simulink model "Micro_Grid_Mains_OFF"  (R2024b)
settings: Solver=VariableStepAuto  StartTime=0.0  StopTime=60*3  RelTol=1e-3
values from neighbouring files (symbols this model uses):
  Pref = 1    [MicroGridParameters.m]
  Ts = 30e-6    (= 3e-05)    [MicroGridParameters.m]
  VDC_Link = 12    [MicroGridParameters.m]
  Vref = 200    [MicroGridParameters.m]
  wref = 1    [MicroGridParameters.m]
libraries: spsSeriesRLCBranchLib x9, spsVoltageMeasurementLib x9, spsThreePhaseVIMeasurementLib x6, spsThreePhaseSeriesRLCBranchLib x5, spsThreePhaseSourceLib x3, spsDiodeLib x3, spsMosfetLib x3, spsPWMGeneratorDCDCLib x3, spsThreePhaseSeriesRLCLoadLib x2, spsBreakerLib x2, spsUniversalBridgeLib x2, slpidlib x2
settings Model: SimulationMode=accelerator  Creator=haima  LastModifiedBy=haima

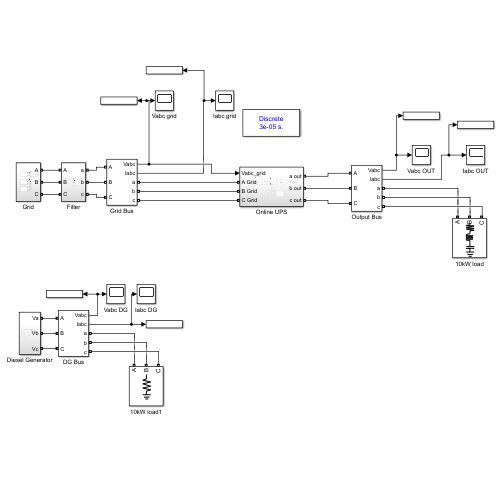
[thumbnail: Simulink's stored preview of the top-level diagram]
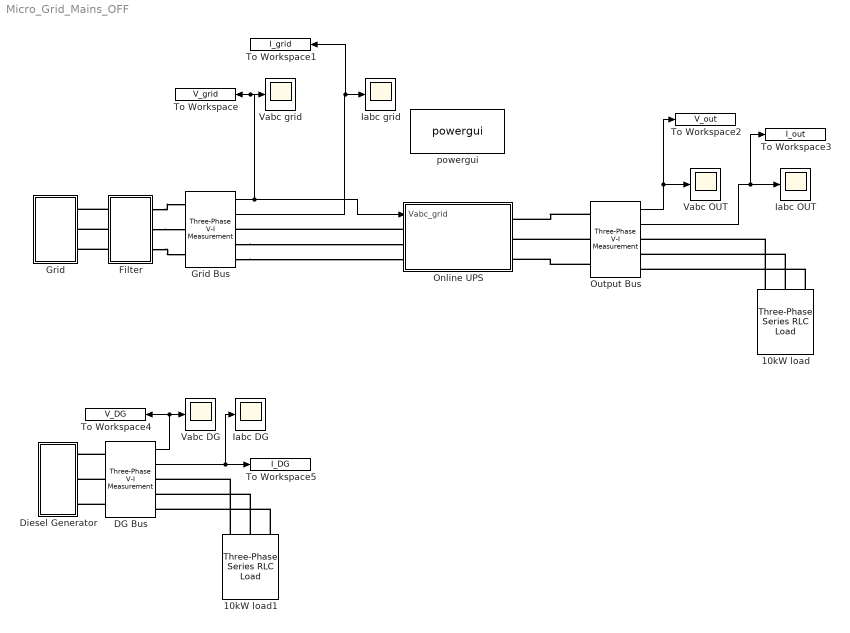
== system Micro_Grid_Mains_OFF ==
  10kW load : spsThreePhaseSeriesRLCLoadLib/Three-Phase Series RLC Load  LConnTagsString=A|B|C  Configuration=Y (grounded)  NominalVoltage=1000  Vabc=[1e3 1e3 1e3]  Vabcp=[1e3 1e3 1e3]  NominalFrequency=50  UnbalancedPower=off  ActivePower=10e3  InductivePower=100  CapacitivePower=100  Pabc=[10e3 9e3 11e3]  QLabc=[100 90 110]  QCabc=[100 90 110]  Pabcp=[10e3 9e3 11e3]  QLabcp=[100 90 110]  QCabcp=[100 90 110]  Measurements=None  LoadType=constant Z
  10kW load1 : spsThreePhaseSeriesRLCLoadLib/Three-Phase Series RLC Load  LConnTagsString=A|B|C  Configuration=Y (grounded)  NominalVoltage=1000  Vabc=[1e3 1e3 1e3]  Vabcp=[1e3 1e3 1e3]  NominalFrequency=50  UnbalancedPower=off  ActivePower=10e3  InductivePower=0  CapacitivePower=0  Pabc=[10e3 9e3 11e3]  QLabc=[100 90 110]  QCabc=[100 90 110]  Pabcp=[10e3 9e3 11e3]  QLabcp=[100 90 110]  QCabcp=[100 90 110]  Measurements=None  LoadType=constant Z
  DG Bus : spsThreePhaseVIMeasurementLib/Three-Phase V-I Measurement  VoltageMeasurement=phase-to-ground  SetLabelV=off  LabelV=Vabc  Vpu=off  VpuLL=off  CurrentMeasurement=yes  SetLabelI=off  LabelI=Iabc  Ipu=off  Pbase=100e6  Vbase=500e3  OutputType=Complex  PhasorSimulation=off  PSBequivalent=0
  Diesel Generator : Subsystem
  Filter : Subsystem
  Grid : Subsystem
  Grid Bus : spsThreePhaseVIMeasurementLib/Three-Phase V-I Measurement  VoltageMeasurement=phase-to-ground  SetLabelV=off  LabelV=Vabc  Vpu=off  VpuLL=off  CurrentMeasurement=yes  SetLabelI=off  LabelI=Iabc  Ipu=off  Pbase=100e6  Vbase=500e3  OutputType=Complex  PhasorSimulation=off  PSBequivalent=0
  Iabc DG : Scope
  Iabc OUT : Scope
  Iabc grid : Scope
  Online UPS : Subsystem
  Output Bus : spsThreePhaseVIMeasurementLib/Three-Phase V-I Measurement  VoltageMeasurement=phase-to-ground  SetLabelV=off  LabelV=Vabc  Vpu=off  VpuLL=off  CurrentMeasurement=yes  SetLabelI=off  LabelI=Iabc  Ipu=off  Pbase=100e6  Vbase=500e3  OutputType=Complex  PhasorSimulation=off  PSBequivalent=0
  To Workspace : ToWorkspace  VariableName=V_grid  SaveFormat=Timeseries  SampleTime=-1
  To Workspace1 : ToWorkspace  VariableName=I_grid  SaveFormat=Timeseries  SampleTime=-1
  To Workspace2 : ToWorkspace  VariableName=V_out  SaveFormat=Timeseries  SampleTime=-1
  To Workspace3 : ToWorkspace  VariableName=I_out  SaveFormat=Timeseries  SampleTime=-1
  To Workspace4 : ToWorkspace  VariableName=V_DG  SaveFormat=Timeseries  SampleTime=-1
  To Workspace5 : ToWorkspace  VariableName=I_DG  SaveFormat=Timeseries  SampleTime=-1
  Vabc DG : Scope
  Vabc OUT : Scope
  Vabc grid : Scope
  powergui : spspowerguiLib/powergui  SimulationMode=Discrete  SampleTime=Ts  frequency=60  Iterations=50  frequencyindice=50  Pbase=100e6  ErrMax=1e-4  UnitsV=kV  UnitsW=MW  buscounter=0  FunctionMessages=off  echomessages=off  EnableUseOfTLC=off  CurrentSourceSwitches=off  DisableSnubberDevices=off  DisableRonSwitches=off  DisableVfSwitches=off  DisplayEquations=off  AutomaticDiscreteSolvers=off  SolverType=Tustin/Backward Euler (TBE)  Interpol=off  ExternalGateDelay=off  methode=off  Ts=100  x0status=blocks  SPID=off  SwTol=0  HookPort=off  NonlinearTolerance=1e-4  nMaxIteration=100  ContinueOnMaxIteration=off  RestoreLinks=warning  ResistiveCurrentMeasurement=off  Frange=[0:2:500]  Ylog=off  Xlog=on  ShowGrid=off  save=off  variable=ZData  structure=Outputs  ZoomFFT=off  StartTime=0.07  cycles=2  DisplayStyle=1  fundamental=50  FreqAxis=on  MaxFrequency=2000  frequencyindicesteady=1  RmsSteady=2  display=off
  wires:
  Grid Bus/1 -> Online UPS/1(Vabc_grid), Vabc grid/1, To Workspace/1
  Grid Bus/2 -> To Workspace1/1, Iabc grid/1
  DG Bus/1 -> Vabc DG/1, To Workspace4/1
  DG Bus/2 -> To Workspace5/1, Iabc DG/1
  Output Bus/1 -> To Workspace2/1, Vabc OUT/1
  Output Bus/2 -> To Workspace3/1, Iabc OUT/1
  connections:
  DG Bus/LConn2 -- Diesel Generator/RConn2
  DG Bus/LConn1 -- Diesel Generator/RConn1
  DG Bus/LConn3 -- Diesel Generator/RConn3
  Output Bus/LConn1 -- Online UPS/RConn1
  Output Bus/LConn2 -- Online UPS/RConn2
  Output Bus/LConn3 -- Online UPS/RConn3
  Filter/LConn1 -- Grid/RConn1
  Filter/LConn2 -- Grid/RConn2
  Filter/LConn3 -- Grid/RConn3
  Filter/RConn2 -- Grid Bus/LConn2
  Filter/RConn1 -- Grid Bus/LConn1
  Filter/RConn3 -- Grid Bus/LConn3
  10kW load/LConn1 -- Output Bus/RConn1
  10kW load/LConn2 -- Output Bus/RConn2
  10kW load/LConn3 -- Output Bus/RConn3
  Online UPS/LConn1 -- Grid Bus/RConn1
  Grid Bus/RConn2 -- Online UPS/LConn2
  Grid Bus/RConn3 -- Online UPS/LConn3
  10kW load1/LConn1 -- DG Bus/RConn1
  10kW load1/LConn2 -- DG Bus/RConn2
  10kW load1/LConn3 -- DG Bus/RConn3

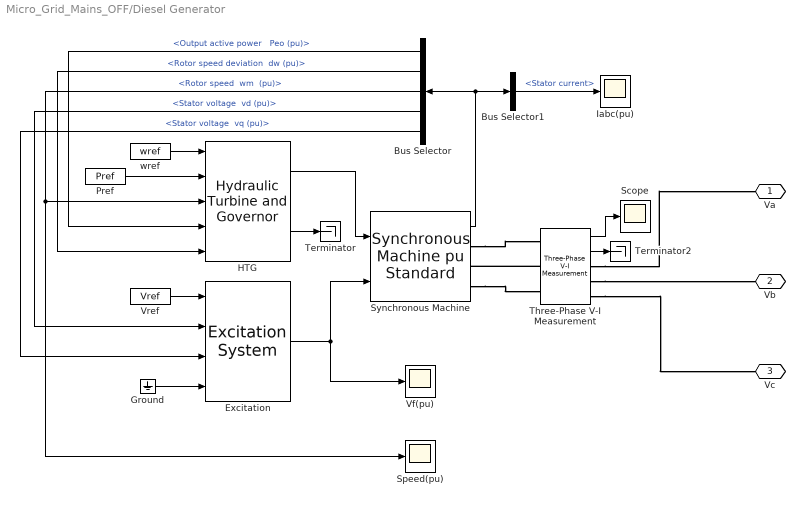
== system Micro_Grid_Mains_OFF/Diesel Generator ==
  Bus Selector : BusSelector  OutputSignals="Output active power   Peo (pu),Mechanical.Rotor speed deviation  dw (pu),Mechanical.Rotor speed  wm  (pu),dq0 components.Stator voltage  vd (pu),dq0 components.Stator voltage  vq (pu)"
  Bus Selector1 : BusSelector  OutputSignals=Stator current
  "Excitation " : spsExcitationSystemLib/Excitation System  tr=20e-3  reg=[ 300, 0.001 ]  exc=[ 1, 0 ]  tgr=[ 0, 0 ]  damp=[ 0.001, 0.1 ]  sat=[ 0, 0 ]  lim=[ -11.5, 11.5, 0 ]  v0="[1.0  1.28]"
  Ground : Ground
  HTG : spsHydraulicTurbineandGovernorLib/Hydraulic Turbine and Governor  sm="[ 10/3  0.07 ]"  gate="[  0.01  0.97518  -0.1  0.1 ]"  reg="[  0.05  1.163  0.105  0  0.01  ]"  hyd="[  0  2.67  ]"  dref=0  po=0.400114
  Iabc(pu) : Scope
  Pref : Constant  Value=Pref
  Scope : Scope
  Speed(pu) : Scope
  "Synchronous Machine " : spsSynchronousMachinepuStandardLib/Synchronous Machine pu Standard  PresetModel=No  MechanicalLoad=Mechanical power Pm  ShowDetailedParameters=on  RotorType=Salient-pole  Units=per unit standard parameters  MeasurementBus=off  NominalParameters=PowerVoltageFrequency  Reactances1=[ 1.81, 0.3, 0.23, 1.76, 0.65, 0.25, 0.15 ]  Reactances2=Reactances  dAxisTimeConstants=Short-circuit  qAxisTimeConstants=Short-circuit  TimeConstants1="[ 4.4849  0.0681  0.1  ]"  TimeConstants2=[ 8.0, 0.03, 1.0, 0.07 ]  TimeConstants3="[  4.49  0.0681  0.0513  ]"  TimeConstants4=[ 8.0, 0.03, 0.3371, 0.0295 ]  TimeConstants5=[ 1.01, 0.053, 0.1 ]  TimeConstants6=[ 1.3201, 0.023, 1.0, 0.07 ]  TimeConstants7=TimeConstants  TimeConstants8=[ 1.3201, 0.0231, 0.3371, 0.0295 ]  StatorResistance=Rs  Mechanical=InertiaFrictionPolePairs  PolePairs=20  InitialConditions=[0 -84.5876 0.2 0.2 0.2 7.01671e-15 -120 120 1.02073]  SetSaturation=on  Saturation=[0.6404,0.7127,0.8441,0.9214,0.9956,1.082,1.19,1.316,1.457;0.7,0.7698,0.8872,0.9466,0.9969,1.046,1.1,1.151,1.201]  LoadFlowParameters=[2 0 0 0 0]  TsPowergui=0  TsBlock=-1  IterativeModel=Trapezoidal non iterative  IterativeDiscreteModel=Trapezoidal non iterative  BusType=PV  Pref=P_total  Qref=0  Qmin=-inf  Qmax=inf  PLF=0  QLF=0
  Terminator : Terminator
  Terminator2 : Terminator
  Three-Phase V-I Measurement : spsThreePhaseVIMeasurementLib/Three-Phase V-I Measurement  VoltageMeasurement=phase-to-ground  SetLabelV=off  LabelV=Vabc  Vpu=off  VpuLL=off  CurrentMeasurement=yes  SetLabelI=off  LabelI=Iabc  Ipu=off  Pbase=100e6  Vbase=500e3  OutputType=Complex  PhasorSimulation=off  PSBequivalent=0
  Vf(pu) : Scope
  Vref : Constant  Value=Vref
  wref : Constant  Value=wref
  Va : PMIOPort  Side=Right
  Vb : PMIOPort  Port=2  Side=Right
  Vc : PMIOPort  Port=3  Side=Right
  wires:
  Pref/1 -> HTG/2
  HTG/1 -> "Synchronous Machine "/1
  Bus Selector/4 -> "Excitation "/2  "<Stator voltage  vd (pu)>"
  HTG/2 -> Terminator/1
  Bus Selector/3 -> Speed(pu)/1, HTG/3  "<Rotor speed  wm  (pu)>"
  wref/1 -> HTG/1
  "Synchronous Machine "/1 -> Bus Selector1/1, Bus Selector/1
  Bus Selector/1 -> HTG/4  "<Output active power   Peo (pu)>"
  Vref/1 -> "Excitation "/1
  Bus Selector1/1 -> Iabc(pu)/1  "<Stator current>"
  Bus Selector/5 -> "Excitation "/3  "<Stator voltage  vq (pu)>"
  "Excitation "/1 -> Vf(pu)/1, "Synchronous Machine "/2
  Bus Selector/2 -> HTG/5  "<Rotor speed deviation  dw (pu)>"
  Ground/1 -> "Excitation "/4
  Three-Phase V-I Measurement/2 -> Terminator2/1
  Three-Phase V-I Measurement/1 -> Scope/1
  connections:
  Three-Phase V-I Measurement/RConn2 -- Vb/RConn1
  Three-Phase V-I Measurement/LConn2 -- "Synchronous Machine "/RConn2
  Three-Phase V-I Measurement/RConn1 -- Va/RConn1
  "Synchronous Machine "/RConn1 -- Three-Phase V-I Measurement/LConn1
  "Synchronous Machine "/RConn3 -- Three-Phase V-I Measurement/LConn3
  Three-Phase V-I Measurement/RConn3 -- Vc/RConn1

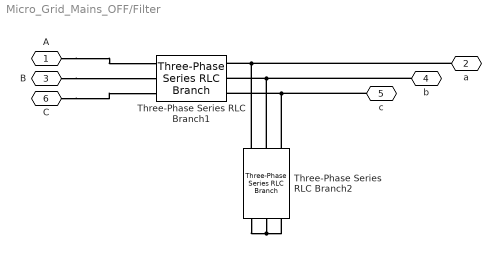
== system Micro_Grid_Mains_OFF/Filter ==
  Three-Phase Series RLC Branch1 : spsThreePhaseSeriesRLCBranchLib/Three-Phase Series RLC Branch  LConnTagsString=A|B|C  RConnTagsString=A|B|C  BranchType=L  Resistance=1  Inductance=500e-6  Capacitance=1e-6  Measurements=None
  Three-Phase Series RLC Branch2 : spsThreePhaseSeriesRLCBranchLib/Three-Phase Series RLC Branch  LConnTagsString=A|B|C  RConnTagsString=A|B|C  BranchType=C  Resistance=1  Inductance=1e-3  Capacitance=100e-6  Measurements=None
  A : PMIOPort  Side=Left
  a : PMIOPort  Port=2  Side=Right
  B : PMIOPort  Port=3  Side=Left
  b : PMIOPort  Port=4  Side=Right
  c : PMIOPort  Port=5  Side=Right
  C : PMIOPort  Port=6  Side=Left
  connections:
  Three-Phase Series RLC Branch2/LConn2 -- Three-Phase Series RLC Branch1/RConn2 -- b/RConn1
  A/RConn1 -- Three-Phase Series RLC Branch1/LConn1
  Three-Phase Series RLC Branch2/RConn1 -- Three-Phase Series RLC Branch2/RConn3 -- Three-Phase Series RLC Branch2/RConn2
  Three-Phase Series RLC Branch2/LConn1 -- Three-Phase Series RLC Branch1/RConn1 -- a/RConn1
  C/RConn1 -- Three-Phase Series RLC Branch1/LConn3
  Three-Phase Series RLC Branch2/LConn3 -- Three-Phase Series RLC Branch1/RConn3 -- c/RConn1
  B/RConn1 -- Three-Phase Series RLC Branch1/LConn2

== system Micro_Grid_Mains_OFF/Grid ==
  three phase power source : spsThreePhaseSourceLib/Three-Phase Source  InternalConnection=Yg  VoltagePhases=off  Voltage=380  PhaseAngle=0  Voltage_phases=[25e3 25e3 25e3]/sqrt(3)  PhaseAngles_phases=[0 -120 +120]  Frequency=50  NonIdealSource=on  SpecifyImpedance=off  Resistance=0.8929  Inductance=16.58e-3  ShortCircuitLevel=100e6  BaseVoltage=380  XRratio=7  BusType=PV  Pref=200e6  Qref=0  Prefabc=[10e3, 10e3, 10e3]  Qrefabc=[0, 0, 0]  Qmin=-inf  Qmax=inf
  three phase power source1 : spsThreePhaseSourceLib/Three-Phase Source  InternalConnection=Yg  VoltagePhases=off  Voltage=380  PhaseAngle=0  Voltage_phases=[25e3 25e3 25e3]/sqrt(3)  PhaseAngles_phases=[0 -120 +120]  Frequency=50  NonIdealSource=on  SpecifyImpedance=off  Resistance=0.8929  Inductance=16.58e-3  ShortCircuitLevel=100e6  BaseVoltage=380  XRratio=7  BusType=PV  Pref=200e6  Qref=0  Prefabc=[10e3, 10e3, 10e3]  Qrefabc=[0, 0, 0]  Qmin=-inf  Qmax=inf
  three phase power source2 : spsThreePhaseSourceLib/Three-Phase Source  InternalConnection=Yg  VoltagePhases=off  Voltage=380  PhaseAngle=0  Voltage_phases=[25e3 25e3 25e3]/sqrt(3)  PhaseAngles_phases=[0 -120 +120]  Frequency=50  NonIdealSource=on  SpecifyImpedance=off  Resistance=0.8929  Inductance=16.58e-3  ShortCircuitLevel=100e6  BaseVoltage=380  XRratio=7  BusType=PV  Pref=200e6  Qref=0  Prefabc=[10e3, 10e3, 10e3]  Qrefabc=[0, 0, 0]  Qmin=-inf  Qmax=inf
  A : PMIOPort  Side=Right
  B : PMIOPort  Port=2  Side=Right
  C : PMIOPort  Port=3  Side=Right
  connections:
  three phase power source/RConn3 -- three phase power source2/RConn3 -- three phase power source1/RConn3 -- C/RConn1
  three phase power source/RConn1 -- A/RConn1 -- three phase power source2/RConn1 -- three phase power source1/RConn1
  three phase power source/RConn2 -- B/RConn1 -- three phase power source2/RConn2 -- three phase power source1/RConn2

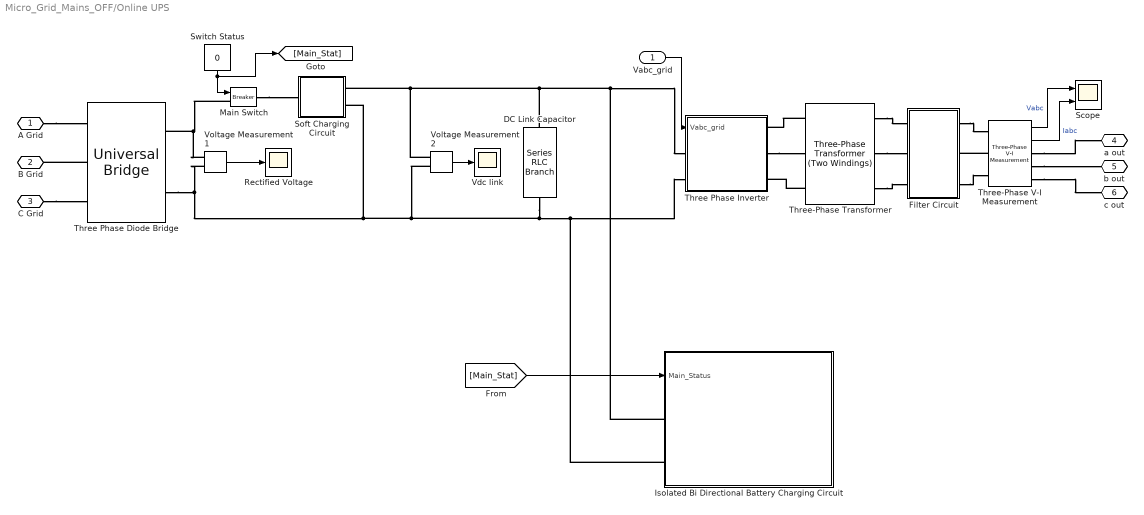
== system Micro_Grid_Mains_OFF/Online UPS ==
  Vabc_grid : Inport
  DC Link Capacitor : spsSeriesRLCBranchLib/Series RLC Branch  LConnTagsString=__new0  RConnTagsString=__new0  BranchType=C  Resistance=1  Inductance=1e-3  SetiL0=off  InitialCurrent=0  Capacitance=50e-6  Setx0=off  InitialVoltage=0  Measurements=None
  Filter Circuit : Subsystem
  Isolated Bi Directional Battery Charging Circuit : Subsystem
  Main Switch : spsBreakerLib/Breaker  InitialState=0  SwitchingTimes="[1/60  5/60]"  External=on  BreakerResistance=0.01  SnubberResistance=inf  SnubberCapacitance=inf  Measurements=None  MoreParameters=on  NoBreakLoop=off
  "Rectified Voltage " : Scope
  Scope : Scope  NumInputPorts=2
  Soft Charging Circuit : Subsystem
  Switch Status : Constant  Value=0
  Three Phase Diode Bridge : spsUniversalBridgeLib/Universal Bridge  Arms=3  SnubberResistance=1e5  SnubberCapacitance=inf  Device=Diodes  Ron=1e-3  Lon=0  ForwardVoltages="[  0  0  ]"  ForwardVoltage=0  GTOparameters=[ 10e-6 , 20e-6 ]  IGBTparameters=[ 1e-6 , 2e-6 ]  Measurements=None  Measurements_2=None  converterType=Rectifier
  Three Phase Inverter : Subsystem
  "Three-Phase Transformer " : spsThreePhaseTransformerTwoWindingsLib/Three-Phase Transformer (Two Windings)  Winding1Connection=Yg  Winding2Connection=Yg  CoreType=Three single-phase transformers  SetSaturation=off  Hysteresis=off  DataFile='hysteresis'  SetInitialFlux=off  Measurements=None  UNITS=pu  NominalPower=[ 500e6 , 50 ]  Winding1=[ 735e3 , 0.002 , 0.08 ]  Winding2=[ 315e3 , 0.002 , 0.08 ]  Rm=500  Lm=500  L0=0.5  Saturation=[ 0,0 ; 0.0024,1.2 ; 1.0,1.52 ]  InitialFluxes=[ 0.8 , -0.8 , 0.7 ]  BreakLoop=off  DiscreteSolver=Trapezoidal iterative  DataType=off  TransfoNumber=1
  Three-Phase V-I Measurement : spsThreePhaseVIMeasurementLib/Three-Phase V-I Measurement  VoltageMeasurement=phase-to-ground  SetLabelV=off  LabelV=Vabc  Vpu=off  VpuLL=off  CurrentMeasurement=yes  SetLabelI=off  LabelI=Iabc  Ipu=off  Pbase=100e6  Vbase=500e3  OutputType=Complex  PhasorSimulation=off  PSBequivalent=0
  Vdc link : Scope
  Voltage Measurement1 : spsVoltageMeasurementLib/Voltage Measurement  PhasorSimulation=off  OutputType=Complex  PSBequivalent=0
  Voltage Measurement2 : spsVoltageMeasurementLib/Voltage Measurement  PhasorSimulation=off  OutputType=Complex  PSBequivalent=0
  A Grid : PMIOPort  Side=Left
  B Grid : PMIOPort  Port=2  Side=Left
  C Grid : PMIOPort  Port=3  Side=Left
  a out : PMIOPort  Port=4  Side=Right
  b out : PMIOPort  Port=5  Side=Right
  c out : PMIOPort  Port=6  Side=Right
  wires:
  Three-Phase V-I Measurement/1 -> Scope/1  "Vabc"
  Voltage Measurement2/1 -> Vdc link/1
  Three-Phase V-I Measurement/2 -> Scope/2  "Iabc"
  Switch Status/1 -> [Main_Stat], Main Switch/1
  [Main_Stat] -> Isolated Bi Directional Battery Charging Circuit/1(Main_Status)
  Voltage Measurement1/1 -> "Rectified Voltage "/1
  Vabc_grid/1 -> Three Phase Inverter/1(Vabc_grid)
  connections:
  "Three-Phase Transformer "/RConn1 -- Filter Circuit/LConn1
  Three-Phase V-I Measurement/LConn2 -- Filter Circuit/RConn2
  Three Phase Inverter/RConn2 -- "Three-Phase Transformer "/LConn2
  C Grid/RConn1 -- Three Phase Diode Bridge/LConn3
  Filter Circuit/RConn3 -- Three-Phase V-I Measurement/LConn3
  Filter Circuit/RConn1 -- Three-Phase V-I Measurement/LConn1
  "Three-Phase Transformer "/LConn1 -- Three Phase Inverter/RConn1
  Three Phase Diode Bridge/RConn1 -- Main Switch/LConn1 -- Voltage Measurement1/LConn1
  "Three-Phase Transformer "/RConn3 -- Filter Circuit/LConn3
  Three-Phase V-I Measurement/RConn3 -- c out/RConn1
  Main Switch/RConn1 -- Soft Charging Circuit/LConn1
  Three-Phase V-I Measurement/RConn1 -- a out/RConn1
  "Three-Phase Transformer "/RConn2 -- Filter Circuit/LConn2
  Three-Phase V-I Measurement/RConn2 -- b out/RConn1
  "Three-Phase Transformer "/LConn3 -- Three Phase Inverter/RConn3
  Three Phase Diode Bridge/LConn2 -- B Grid/RConn1
  A Grid/RConn1 -- Three Phase Diode Bridge/LConn1
  Voltage Measurement2/LConn1 -- Three Phase Inverter/LConn1 -- Isolated Bi Directional Battery Charging Circuit/LConn1 -- DC Link Capacitor/LConn1 -- Soft Charging Circuit/RConn1
  DC Link Capacitor/RConn1 -- Three Phase Inverter/LConn2 -- Isolated Bi Directional Battery Charging Circuit/LConn2 -- Voltage Measurement2/LConn2 -- Three Phase Diode Bridge/RConn2 -- Voltage Measurement1/LConn2 -- Soft Charging Circuit/RConn2

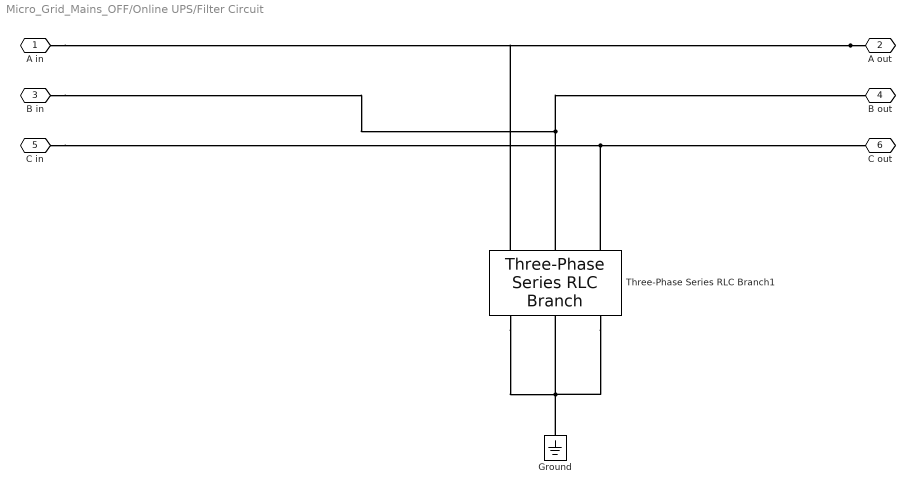
== system Micro_Grid_Mains_OFF/Online UPS/Filter Circuit ==
  Ground : spsGroundLib/Ground  LConnTagsString=a
  Three-Phase Series RLC Branch1 : spsThreePhaseSeriesRLCBranchLib/Three-Phase Series RLC Branch  LConnTagsString=A|B|C  RConnTagsString=A|B|C  BranchType=C  Resistance=1  Inductance=1e-3  Capacitance=50e-6  Measurements=None
  A in : PMIOPort  Side=Left
  A out : PMIOPort  Port=2  Side=Right
  B in : PMIOPort  Port=3  Side=Left
  B out : PMIOPort  Port=4  Side=Right
  C in : PMIOPort  Port=5  Side=Left
  C out : PMIOPort  Port=6  Side=Right
  connections:
  A out/RConn1 -- Three-Phase Series RLC Branch1/LConn1 -- A in/RConn1
  Three-Phase Series RLC Branch1/LConn2 -- B in/RConn1 -- B out/RConn1
  Three-Phase Series RLC Branch1/LConn3 -- C in/RConn1 -- C out/RConn1
  Ground/LConn1 -- Three-Phase Series RLC Branch1/RConn3 -- Three-Phase Series RLC Branch1/RConn1 -- Three-Phase Series RLC Branch1/RConn2

== system Micro_Grid_Mains_OFF/Online UPS/Isolated Bi Directional Battery Charging Circuit ==
  Main_Status : Inport
  Boost Converter : Subsystem
  DC Voltage Source : spsDCVoltageSourceLib/DC Voltage Source  Amplitude=VDC_Link  Measurements=None
  Terminator : Terminator
  + : PMIOPort  Side=Left
  - : PMIOPort  Port=2  Side=Left
  wires:
  Main_Status/1 -> Terminator/1
  connections:
  Boost Converter/RConn2 -- DC Voltage Source/LConn1
  DC Voltage Source/RConn1 -- Boost Converter/RConn1
  Boost Converter/LConn1 -- +/RConn1
  Boost Converter/LConn2 -- -/RConn1

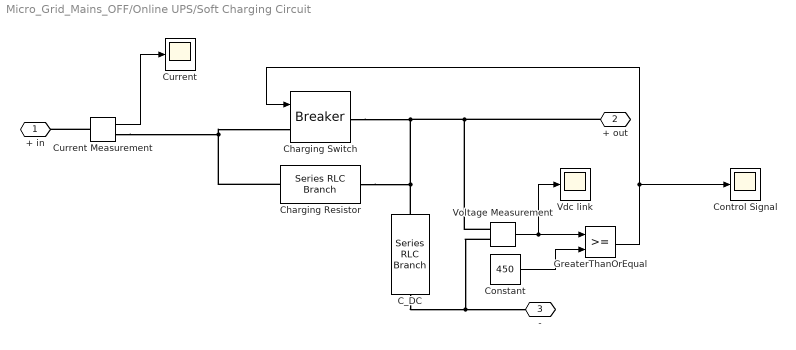
== system Micro_Grid_Mains_OFF/Online UPS/Soft Charging Circuit ==
  C_DC : spsSeriesRLCBranchLib/Series RLC Branch  LConnTagsString=__new0  RConnTagsString=__new0  BranchType=C  Resistance=1  Inductance=1e-3  SetiL0=off  InitialCurrent=0  Capacitance=6.4e-3  Setx0=off  InitialVoltage=0  Measurements=None
  Charging Resistor : spsSeriesRLCBranchLib/Series RLC Branch  LConnTagsString=__new0  RConnTagsString=__new0  BranchType=R  Resistance=10  Inductance=16.8e-3  SetiL0=off  InitialCurrent=0  Capacitance=1e-6  Setx0=off  InitialVoltage=0  Measurements=None
  Charging Switch : spsBreakerLib/Breaker  InitialState=0  SwitchingTimes="[1/60  5/60]"  External=on  BreakerResistance=0.01  SnubberResistance=inf  SnubberCapacitance=inf  Measurements=None  MoreParameters=on  NoBreakLoop=off
  Constant : Constant  Value=450
  Control Signal : Scope
  Current : Scope
  Current Measurement : spsCurrentMeasurementLib/Current Measurement  PhasorSimulation=off  OutputType=Complex  PSBequivalent=0
  GreaterThanOrEqual : RelationalOperator  OutDataTypeStr=boolean  RndMeth=Simplest  InputSameDT=off
  Vdc link : Scope
  Voltage Measurement : spsVoltageMeasurementLib/Voltage Measurement  PhasorSimulation=off  OutputType=Complex  PSBequivalent=0
  + in : PMIOPort  Side=Left
  + out : PMIOPort  Port=2  Side=Right
  - : PMIOPort  Port=3  Side=Right
  wires:
  Voltage Measurement/1 -> Vdc link/1, GreaterThanOrEqual/1
  Constant/1 -> GreaterThanOrEqual/2
  GreaterThanOrEqual/1 -> Control Signal/1, Charging Switch/1
  Current Measurement/1 -> Current/1
  connections:
  Charging Resistor/LConn1 -- Current Measurement/RConn1 -- Charging Switch/LConn1
  Charging Switch/RConn1 -- + out/RConn1 -- Voltage Measurement/LConn1 -- C_DC/LConn1 -- Charging Resistor/RConn1
  C_DC/RConn1 -- Voltage Measurement/LConn2 -- -/RConn1
  Current Measurement/LConn1 -- + in/RConn1

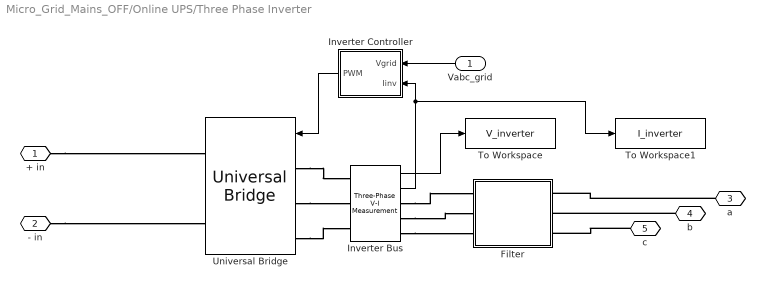
== system Micro_Grid_Mains_OFF/Online UPS/Three Phase Inverter ==
  Vabc_grid : Inport
  Filter : Subsystem
  Inverter Controller : Subsystem  mask(Direct-Quadrature Synchronous Reference Frame Controller){Id=100, Iq=0, VDC=800, f=50, fsw=10000, L=1000e-6, kp=5, ki=5000}
      mask prompts: Id "Active Current (A)"; Iq "Reactive Current (A)"; VDC "DC Link Voltage (V)"; f "Grid Frequency (Hz)"; fsw "Switching Frequency (Hz)"; L "Filter Inductance (H)"; kp "Proportional Gain"; ki "Integral Gain"
      mask help:
      | Developed by Rodney Tan (PhD)
      | Version 1.0 (Nov 2021)
      |
      | This model demonstrate the operation of 3 phase grid connected inverter using Direct-Quadrature Synchronous Reference Frame Control.
      |
      | SPWM is use to switch the IGBT inverter bridge.
      |
      | The controller allows user to set the DC link voltage, active and reactive current for the inverter to be injected to the grid.
      |
      | The scope monitor the grid inverter output voltage and current waveform.
      |
      | The display monitor the active and reactive power injected to the grid.
      mask DialogControl Container3 Prompt: PI Controller Setting
  Inverter Bus : spsThreePhaseVIMeasurementLib/Three-Phase V-I Measurement  VoltageMeasurement=phase-to-phase  SetLabelV=off  LabelV=Vabc  Vpu=off  VpuLL=off  CurrentMeasurement=yes  SetLabelI=off  LabelI=Iabc  Ipu=off  Pbase=100e6  Vbase=500e3  OutputType=Complex  PhasorSimulation=off  PSBequivalent=0
  To Workspace : ToWorkspace  VariableName=V_inverter  SaveFormat=Timeseries  SampleTime=-1
  To Workspace1 : ToWorkspace  VariableName=I_inverter  SaveFormat=Timeseries  SampleTime=-1
  Universal Bridge : spsUniversalBridgeLib/Universal Bridge  Arms=3  SnubberResistance=1e5  SnubberCapacitance=inf  Device=IGBT / Diodes  Ron=1e-3  Lon=0  ForwardVoltages="[  0  0  ]"  ForwardVoltage=0  GTOparameters=[ 10e-6 , 20e-6 ]  IGBTparameters=[ 1e-6 , 2e-6 ]  Measurements=None  Measurements_2=None  converterType=Rectifier
  + in : PMIOPort  Side=Left
  - in : PMIOPort  Port=2  Side=Left
  a : PMIOPort  Port=3  Side=Right
  b : PMIOPort  Port=4  Side=Right
  c : PMIOPort  Port=5  Side=Right
  wires:
  Inverter Controller/1(PWM) -> Universal Bridge/1
  Inverter Bus/2 -> Inverter Controller/2(Iinv), To Workspace1/1
  Vabc_grid/1 -> Inverter Controller/1(Vgrid)
  Inverter Bus/1 -> To Workspace/1
  connections:
  + in/RConn1 -- Universal Bridge/RConn1
  - in/RConn1 -- Universal Bridge/RConn2
  Universal Bridge/LConn1 -- Inverter Bus/LConn1
  Universal Bridge/LConn2 -- Inverter Bus/LConn2
  Universal Bridge/LConn3 -- Inverter Bus/LConn3
  Inverter Bus/RConn1 -- Filter/LConn1
  a/RConn1 -- Filter/RConn1
  Inverter Bus/RConn2 -- Filter/LConn2
  b/RConn1 -- Filter/RConn2
  c/RConn1 -- Filter/RConn3
  Inverter Bus/RConn3 -- Filter/LConn3

== system Micro_Grid_Mains_OFF/Online UPS/Isolated Bi Directional Battery Charging Circuit/Boost Converter ==
  Boost Converter : Subsystem
  Boost Converter1 : Subsystem
  Boost Converter2 : Subsystem
  + out : PMIOPort  Side=Left
  - out : PMIOPort  Port=2  Side=Left
  + in : PMIOPort  Port=3  Side=Right
  - in : PMIOPort  Port=4  Side=Right
  connections:
  Boost Converter1/LConn1 -- Boost Converter/RConn1
  Boost Converter1/LConn2 -- Boost Converter/RConn2
  + in/RConn1 -- Boost Converter1/RConn1
  Boost Converter2/RConn1 -- Boost Converter/LConn1
  Boost Converter2/RConn2 -- Boost Converter/LConn2
  - out/RConn1 -- Boost Converter2/LConn2
  + out/RConn1 -- Boost Converter2/LConn1
  - in/RConn1 -- Boost Converter1/RConn2

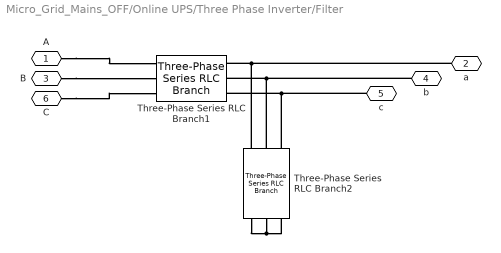
== system Micro_Grid_Mains_OFF/Online UPS/Three Phase Inverter/Filter ==
  Three-Phase Series RLC Branch1 : spsThreePhaseSeriesRLCBranchLib/Three-Phase Series RLC Branch  LConnTagsString=A|B|C  RConnTagsString=A|B|C  BranchType=L  Resistance=1  Inductance=500e-6  Capacitance=1e-6  Measurements=None
  Three-Phase Series RLC Branch2 : spsThreePhaseSeriesRLCBranchLib/Three-Phase Series RLC Branch  LConnTagsString=A|B|C  RConnTagsString=A|B|C  BranchType=C  Resistance=1  Inductance=1e-3  Capacitance=100e-6  Measurements=None
  A : PMIOPort  Side=Left
  a : PMIOPort  Port=2  Side=Right
  B : PMIOPort  Port=3  Side=Left
  b : PMIOPort  Port=4  Side=Right
  c : PMIOPort  Port=5  Side=Right
  C : PMIOPort  Port=6  Side=Left
  connections:
  Three-Phase Series RLC Branch2/LConn2 -- b/RConn1 -- Three-Phase Series RLC Branch1/RConn2
  A/RConn1 -- Three-Phase Series RLC Branch1/LConn1
  Three-Phase Series RLC Branch2/RConn1 -- Three-Phase Series RLC Branch2/RConn2 -- Three-Phase Series RLC Branch2/RConn3
  Three-Phase Series RLC Branch2/LConn1 -- a/RConn1 -- Three-Phase Series RLC Branch1/RConn1
  C/RConn1 -- Three-Phase Series RLC Branch1/LConn3
  Three-Phase Series RLC Branch2/LConn3 -- c/RConn1 -- Three-Phase Series RLC Branch1/RConn3
  B/RConn1 -- Three-Phase Series RLC Branch1/LConn2

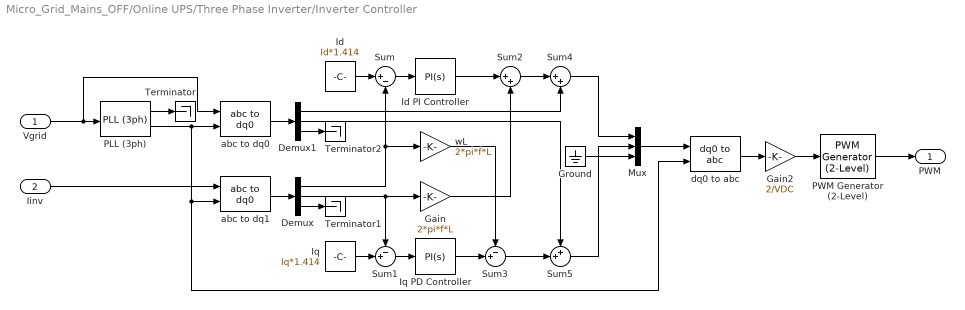
== system Micro_Grid_Mains_OFF/Online UPS/Three Phase Inverter/Inverter Controller ==
  Vgrid : Inport
  Iinv : Inport  Port=2
  Demux : Demux  Outputs=3
  Demux1 : Demux  Outputs=3
  Gain : Gain  Gain=2*pi*f*L
  Gain2 : Gain  Gain=2/VDC
  Ground : Ground
  Id : Constant  Value=Id*1.414
  Id PI Controller : slpidlib/PID Controller  Controller=PI  Form=Parallel  TimeDomain=Continuous-time  UseExternalTs=off  SampleTime=-1  IntegratorMethod=Forward Euler  FilterMethod=Forward Euler  ControllerParametersSource=internal  P=kp  I=ki  UseKiTs=off  D=0  UseExternalDerivativeSource=off  N=100  UseFilter=on  TunerSelectOption=Transfer Function Based (PID Tuner App)  InitialConditionSource=internal  InitialConditionForIntegrator=0  InitialConditionForFilter=0  DifferentiatorICPrevScaledInput=0  ExternalReset=none  TrackingMode=off  Kt=1  LimitOutput=off  SatLimitsSource=internal  UpperSaturationLimit=inf  LowerSaturationLimit=-inf  LinearizeAsGain=on  AntiWindupMode=none  Kb=1  LimitIntegrator=off  UpperIntegratorSaturationLimit=inf  LowerIntegratorSaturationLimit=-inf  POutMin=[]  POutMax=[]  IOutMin=[]  IOutMax=[]  DOutMin=[]  DOutMax=[]  NOutMin=[]  NOutMax=[]  SumOutMin=[]  SumOutMax=[]  SaturationOutMin=[]  SaturationOutMax=[]  PParamMin=[]  PParamMax=[]  IParamMin=[]  IParamMax=[]  DParamMin=[]  DParamMax=[]  NParamMin=[]  NParamMax=[]  KbParamMin=[]  KbParamMax=[]  KtParamMin=[]  KtParamMax=[]  KbOutMin=[]  KbOutMax=[]  KtOutMin=[]  KtOutMax=[]  IntegratorOutMin=[]  IntegratorOutMax=[]  FilterOutMin=[]  FilterOutMax=[]  SumI1OutMin=[]  SumI1OutMax=[]  SumI2OutMin=[]  SumI2OutMax=[]  SumI3OutMin=[]  SumI3OutMax=[]  SumI4OutMin=[]  SumI4OutMax=[]  SumDOutMin=[]  SumDOutMax=[]  DifferentiatorOutMin=[]  DifferentiatorOutMax=[]  FilterDiffOutCoefMin=[]  FilterDiffOutCoefMax=[]  ReciprocalOutMin=[]  ReciprocalOutMax=[]  SumDenOutMin=[]  SumDenOutMax=[]  SumNumOutMin=[]  SumNumOutMax=[]  DivideOutMin=[]  DivideOutMax=[]  UdiffTsProdOutMin=[]  UdiffTsProdOutMax=[]  NTsProdOutMin=[]  NTsProdOutMax=[]  UintegralTsProdOutMin=[]  UintegralTsProdOutMax=[]  UngainTsProdOutMin=[]  UngainTsProdOutMax=[]  ClampingZeroOutDataTypeStr=Inherit: Inherit via back propagation  ClampingZeroOutMin=[]  ClampingZeroOutMax=[]  FilterDenConstantOutDataTypeStr=Inherit: Inherit via back propagation  FilterDenConstantOutMin=[]  FilterDenConstantOutMax=[]  PCopyOutDataTypeStr=Inherit: Inherit via back propagation  PCopyOutMin=[]  PCopyOutMax=[]  NCopyOutDataTypeStr=Inherit: Inherit via back propagation  NCopyOutMin=[]  NCopyOutMax=[]  IntegratorContinuousStateAttributes=''  IntegratorStateMustResolveToSignalObject=off  IntegratorRTWStateStorageClass=Auto  FilterContinuousStateAttributes=''  FilterStateMustResolveToSignalObject=off  FilterRTWStateStorageClass=Auto  ParallelPVariant=InternalParameters  IdealPVariant=Disabled  IVariant=InternalParameters  DVariant=Disabled  IntegratorVariant=Continuous  SatVariant=Disabled  AWVariant=Passthrough  PCopyVariant=Disabled  TRVariant=Disabled  FdbkBlocksVariant=Forward  IdealPFdbkVariant=Disabled  SatFdbkVariant=Disabled  DerivativeFilterVariant=Disabled  NVariant=Disabled  NCopyVariant=Disabled_SignalSpec  FilterICVariant=Disabled  IntegratorICVariant=InternalICs  ExternalResetVariant=Disabled  TRSumVariant=Passthrough  SumFdbkVariant=Disabled  SumVariant=Sum_PI  TsampFilterVariant=InternalTs  TsampNgainVariant=Passthrough  TsampIntegralVariant=Disabled_SignalSpec  ExternalSaturationOutDataTypeStr=Inherit: Same as second input  DerivativeSourceVariant=Disabled  PreIntVariant=InternalPreInt
  Iq : Constant  Value=Iq*1.414
  Iq PD Controller : slpidlib/PID Controller  Controller=PI  Form=Parallel  TimeDomain=Continuous-time  UseExternalTs=off  SampleTime=-1  IntegratorMethod=Forward Euler  FilterMethod=Forward Euler  ControllerParametersSource=internal  P=kp  I=ki  UseKiTs=off  D=0  UseExternalDerivativeSource=off  N=100  UseFilter=on  TunerSelectOption=Transfer Function Based (PID Tuner App)  InitialConditionSource=internal  InitialConditionForIntegrator=0  InitialConditionForFilter=0  DifferentiatorICPrevScaledInput=0  ExternalReset=none  TrackingMode=off  Kt=1  LimitOutput=off  SatLimitsSource=internal  UpperSaturationLimit=inf  LowerSaturationLimit=-inf  LinearizeAsGain=on  AntiWindupMode=none  Kb=1  LimitIntegrator=off  UpperIntegratorSaturationLimit=inf  LowerIntegratorSaturationLimit=-inf  POutMin=[]  POutMax=[]  IOutMin=[]  IOutMax=[]  DOutMin=[]  DOutMax=[]  NOutMin=[]  NOutMax=[]  SumOutMin=[]  SumOutMax=[]  SaturationOutMin=[]  SaturationOutMax=[]  PParamMin=[]  PParamMax=[]  IParamMin=[]  IParamMax=[]  DParamMin=[]  DParamMax=[]  NParamMin=[]  NParamMax=[]  KbParamMin=[]  KbParamMax=[]  KtParamMin=[]  KtParamMax=[]  KbOutMin=[]  KbOutMax=[]  KtOutMin=[]  KtOutMax=[]  IntegratorOutMin=[]  IntegratorOutMax=[]  FilterOutMin=[]  FilterOutMax=[]  SumI1OutMin=[]  SumI1OutMax=[]  SumI2OutMin=[]  SumI2OutMax=[]  SumI3OutMin=[]  SumI3OutMax=[]  SumI4OutMin=[]  SumI4OutMax=[]  SumDOutMin=[]  SumDOutMax=[]  DifferentiatorOutMin=[]  DifferentiatorOutMax=[]  FilterDiffOutCoefMin=[]  FilterDiffOutCoefMax=[]  ReciprocalOutMin=[]  ReciprocalOutMax=[]  SumDenOutMin=[]  SumDenOutMax=[]  SumNumOutMin=[]  SumNumOutMax=[]  DivideOutMin=[]  DivideOutMax=[]  UdiffTsProdOutMin=[]  UdiffTsProdOutMax=[]  NTsProdOutMin=[]  NTsProdOutMax=[]  UintegralTsProdOutMin=[]  UintegralTsProdOutMax=[]  UngainTsProdOutMin=[]  UngainTsProdOutMax=[]  ClampingZeroOutDataTypeStr=Inherit: Inherit via back propagation  ClampingZeroOutMin=[]  ClampingZeroOutMax=[]  FilterDenConstantOutDataTypeStr=Inherit: Inherit via back propagation  FilterDenConstantOutMin=[]  FilterDenConstantOutMax=[]  PCopyOutDataTypeStr=Inherit: Inherit via back propagation  PCopyOutMin=[]  PCopyOutMax=[]  NCopyOutDataTypeStr=Inherit: Inherit via back propagation  NCopyOutMin=[]  NCopyOutMax=[]  IntegratorContinuousStateAttributes=''  IntegratorStateMustResolveToSignalObject=off  IntegratorRTWStateStorageClass=Auto  FilterContinuousStateAttributes=''  FilterStateMustResolveToSignalObject=off  FilterRTWStateStorageClass=Auto  ParallelPVariant=InternalParameters  IdealPVariant=Disabled  IVariant=InternalParameters  DVariant=Disabled  IntegratorVariant=Continuous  SatVariant=Disabled  AWVariant=Passthrough  PCopyVariant=Disabled  TRVariant=Disabled  FdbkBlocksVariant=Forward  IdealPFdbkVariant=Disabled  SatFdbkVariant=Disabled  DerivativeFilterVariant=Disabled  NVariant=Disabled  NCopyVariant=Disabled_SignalSpec  FilterICVariant=Disabled  IntegratorICVariant=InternalICs  ExternalResetVariant=Disabled  TRSumVariant=Passthrough  SumFdbkVariant=Disabled  SumVariant=Sum_PI  TsampFilterVariant=InternalTs  TsampNgainVariant=Passthrough  TsampIntegralVariant=Disabled_SignalSpec  ExternalSaturationOutDataTypeStr=Inherit: Same as second input  DerivativeSourceVariant=Disabled  PreIntVariant=InternalPreInt
  Mux : Mux  Inputs=3
  PLL (3ph) : spsPLL3phLib/PLL (3ph)  Fmin=45  Par_Init=[0, f]  ParK=[180, 3200, 1]  TcD=1e-4  MaxRateChangeFreq=12  FilterCutOffFreq=25  Ts=0  AGC=on
  PWM Generator (2-Level) : spsPWMGenerator2LevelLib/PWM Generator (2-Level)  ModulatorType=Three-phase bridge (6 pulses)  ModulatorMode=Unsynchronized  Fc=fsw  Pc=0  nF=27  MinMax="[ -1  1 ]"  SamplingTechnique=Natural  ModulatingSignals=off  m=0.8  Freq=60  Phase=0  Ts=0  ShowCarrierOutport=off
  Sum : Sum  Inputs=|+-
  Sum1 : Sum  Inputs=-+|
  Sum2 : Sum  Inputs=|++
  Sum3 : Sum  Inputs=-+|
  Sum4 : Sum  Inputs=|++
  Sum5 : Sum  Inputs=++|
  Terminator : Terminator
  Terminator1 : Terminator
  Terminator2 : Terminator
  abc to dq0 : spsabctodq0Lib/abc to dq0  Alignment=90 degrees behind phase A axis
  abc to dq1 : spsabctodq0Lib/abc to dq0  Alignment=90 degrees behind phase A axis
  dq0 to abc : spsdq0toabcLib/dq0 to abc  Alignment=90 degrees behind phase A axis
  wL : Gain  Gain=2*pi*f*L
  PWM : Outport
  wires:
  PWM Generator (2-Level)/1 -> PWM/1
  Id PI Controller/1 -> Sum2/1
  Gain2/1 -> PWM Generator (2-Level)/1
  abc to dq0/1 -> Demux1/1
  Ground/1 -> Mux/3
  wL/1 -> Sum3/1
  PLL (3ph)/2 -> dq0 to abc/2, abc to dq1/2, abc to dq0/2
  Gain/1 -> Sum2/2
  dq0 to abc/1 -> Gain2/1
  Demux1/1 -> Sum4/2
  Sum1/1 -> Iq PD Controller/1
  Vgrid/1 -> abc to dq0/1, PLL (3ph)/1
  Sum/1 -> Id PI Controller/1
  Demux1/3 -> Terminator2/1
  abc to dq1/1 -> Demux/1
  Sum2/1 -> Sum4/1
  Mux/1 -> dq0 to abc/1
  Demux1/2 -> Sum5/1
  Sum3/1 -> Sum5/2
  Iq/1 -> Sum1/2
  Sum5/1 -> Mux/2
  Demux/1 -> wL/1, Sum/2
  Iq PD Controller/1 -> Sum3/2
  Sum4/1 -> Mux/1
  Id/1 -> Sum/1
  PLL (3ph)/1 -> Terminator/1
  Demux/2 -> Sum1/1, Gain/1
  Demux/3 -> Terminator1/1
  Iinv/1 -> abc to dq1/1

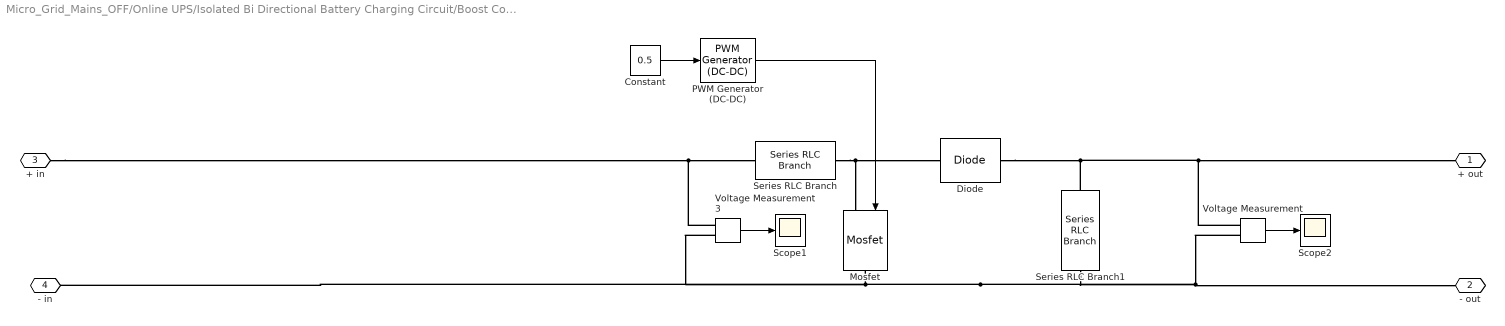
== system Micro_Grid_Mains_OFF/Online UPS/Isolated Bi Directional Battery Charging Circuit/Boost Converter/Boost Converter ==
  Constant : Constant  Value=0.5
  Diode : spsDiodeLib/Diode  Ron=0.001  Lon=0  Vf=0  IC=0  UseSnubber=0  Rs=inf  Cs=inf  Measurements=off
  Mosfet : spsMosfetLib/Mosfet  Ron=0.1  Lon=0  Rd=0.01  Vfd=0  IC=0  Rs=1e10  Cs=inf  Measurements=off
  PWM Generator (DC-DC) : spsPWMGeneratorDCDCLib/PWM Generator (DC-DC)  Fsw=21.23568945621356e3  Ts=0
  Scope1 : Scope
  Scope2 : Scope
  Series RLC Branch : spsSeriesRLCBranchLib/Series RLC Branch  LConnTagsString=__new0  RConnTagsString=__new0  BranchType=RL  Resistance=1e-6  Inductance=250e-5  SetiL0=off  InitialCurrent=0  Capacitance=1e-6  Setx0=off  InitialVoltage=0  Measurements=None
  Series RLC Branch1 : spsSeriesRLCBranchLib/Series RLC Branch  LConnTagsString=__new0  RConnTagsString=__new0  BranchType=C  Resistance=1  Inductance=1e-3  SetiL0=off  InitialCurrent=0  Capacitance=20e-5  Setx0=off  InitialVoltage=0  Measurements=None
  Voltage Measurement : spsVoltageMeasurementLib/Voltage Measurement  PhasorSimulation=off  OutputType=Complex  PSBequivalent=0
  Voltage Measurement3 : spsVoltageMeasurementLib/Voltage Measurement  PhasorSimulation=off  OutputType=Complex  PSBequivalent=0
  + out : PMIOPort  Side=Left
  - out : PMIOPort  Port=2  Side=Left
  + in : PMIOPort  Port=3  Side=Right
  - in : PMIOPort  Port=4  Side=Right
  wires:
  Voltage Measurement/1 -> Scope2/1
  Voltage Measurement3/1 -> Scope1/1
  Constant/1 -> PWM Generator (DC-DC)/1
  PWM Generator (DC-DC)/1 -> Mosfet/1
  connections:
  Voltage Measurement/LConn1 -- + out/RConn1 -- Series RLC Branch1/LConn1 -- Diode/RConn1
  Voltage Measurement3/LConn1 -- + in/RConn1 -- Series RLC Branch/LConn1
  Voltage Measurement/LConn2 -- - out/RConn1 -- Series RLC Branch1/RConn1 -- Voltage Measurement3/LConn2 -- - in/RConn1 -- Mosfet/RConn1
  Series RLC Branch/RConn1 -- Diode/LConn1 -- Mosfet/LConn1

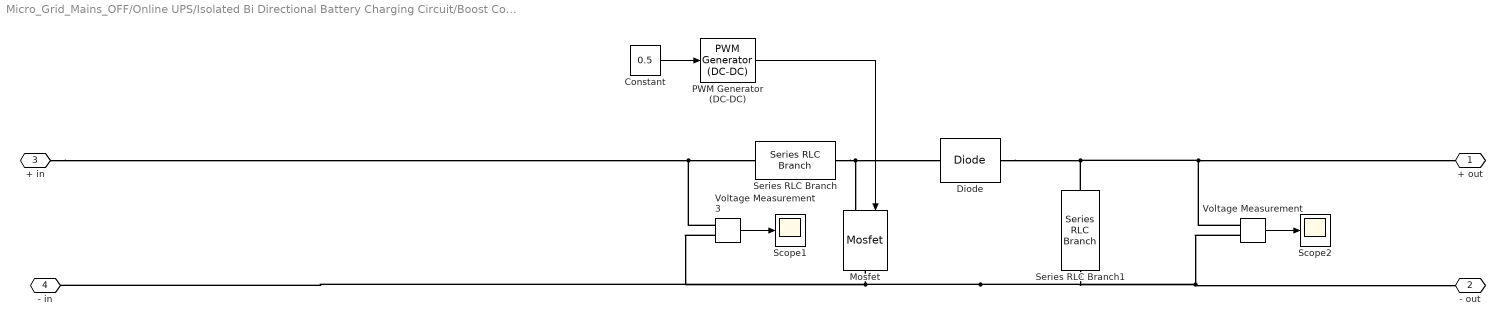
== system Micro_Grid_Mains_OFF/Online UPS/Isolated Bi Directional Battery Charging Circuit/Boost Converter/Boost Converter1 ==
  Constant : Constant  Value=0.5
  Diode : spsDiodeLib/Diode  Ron=0.001  Lon=0  Vf=0  IC=0  UseSnubber=0  Rs=inf  Cs=inf  Measurements=off
  Mosfet : spsMosfetLib/Mosfet  Ron=0.1  Lon=0  Rd=0.01  Vfd=0  IC=0  Rs=1e10  Cs=inf  Measurements=off
  PWM Generator (DC-DC) : spsPWMGeneratorDCDCLib/PWM Generator (DC-DC)  Fsw=21.23568945621356e3  Ts=0
  Scope1 : Scope
  Scope2 : Scope
  Series RLC Branch : spsSeriesRLCBranchLib/Series RLC Branch  LConnTagsString=__new0  RConnTagsString=__new0  BranchType=RL  Resistance=1e-6  Inductance=250e-5  SetiL0=off  InitialCurrent=0  Capacitance=1e-6  Setx0=off  InitialVoltage=0  Measurements=None
  Series RLC Branch1 : spsSeriesRLCBranchLib/Series RLC Branch  LConnTagsString=__new0  RConnTagsString=__new0  BranchType=C  Resistance=1  Inductance=1e-3  SetiL0=off  InitialCurrent=0  Capacitance=20e-5  Setx0=off  InitialVoltage=0  Measurements=None
  Voltage Measurement : spsVoltageMeasurementLib/Voltage Measurement  PhasorSimulation=off  OutputType=Complex  PSBequivalent=0
  Voltage Measurement3 : spsVoltageMeasurementLib/Voltage Measurement  PhasorSimulation=off  OutputType=Complex  PSBequivalent=0
  + out : PMIOPort  Side=Left
  - out : PMIOPort  Port=2  Side=Left
  + in : PMIOPort  Port=3  Side=Right
  - in : PMIOPort  Port=4  Side=Right
  wires:
  Voltage Measurement/1 -> Scope2/1
  Voltage Measurement3/1 -> Scope1/1
  Constant/1 -> PWM Generator (DC-DC)/1
  PWM Generator (DC-DC)/1 -> Mosfet/1
  connections:
  Voltage Measurement/LConn1 -- + out/RConn1 -- Series RLC Branch1/LConn1 -- Diode/RConn1
  Voltage Measurement3/LConn1 -- + in/RConn1 -- Series RLC Branch/LConn1
  Voltage Measurement/LConn2 -- - out/RConn1 -- Series RLC Branch1/RConn1 -- Voltage Measurement3/LConn2 -- - in/RConn1 -- Mosfet/RConn1
  Series RLC Branch/RConn1 -- Diode/LConn1 -- Mosfet/LConn1

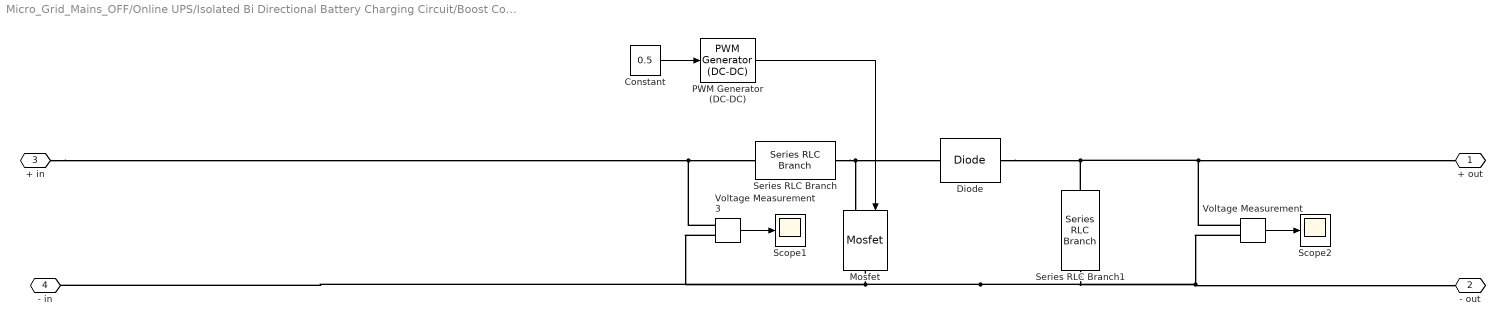
== system Micro_Grid_Mains_OFF/Online UPS/Isolated Bi Directional Battery Charging Circuit/Boost Converter/Boost Converter2 ==
  Constant : Constant  Value=0.5
  Diode : spsDiodeLib/Diode  Ron=0.001  Lon=0  Vf=0  IC=0  UseSnubber=0  Rs=inf  Cs=inf  Measurements=off
  Mosfet : spsMosfetLib/Mosfet  Ron=0.1  Lon=0  Rd=0.01  Vfd=0  IC=0  Rs=1e10  Cs=inf  Measurements=off
  PWM Generator (DC-DC) : spsPWMGeneratorDCDCLib/PWM Generator (DC-DC)  Fsw=21.23568945621356e3  Ts=0
  Scope1 : Scope
  Scope2 : Scope
  Series RLC Branch : spsSeriesRLCBranchLib/Series RLC Branch  LConnTagsString=__new0  RConnTagsString=__new0  BranchType=RL  Resistance=1e-6  Inductance=250e-5  SetiL0=off  InitialCurrent=0  Capacitance=1e-6  Setx0=off  InitialVoltage=0  Measurements=None
  Series RLC Branch1 : spsSeriesRLCBranchLib/Series RLC Branch  LConnTagsString=__new0  RConnTagsString=__new0  BranchType=C  Resistance=1  Inductance=1e-3  SetiL0=off  InitialCurrent=0  Capacitance=20e-5  Setx0=off  InitialVoltage=0  Measurements=None
  Voltage Measurement : spsVoltageMeasurementLib/Voltage Measurement  PhasorSimulation=off  OutputType=Complex  PSBequivalent=0
  Voltage Measurement3 : spsVoltageMeasurementLib/Voltage Measurement  PhasorSimulation=off  OutputType=Complex  PSBequivalent=0
  + out : PMIOPort  Side=Left
  - out : PMIOPort  Port=2  Side=Left
  + in : PMIOPort  Port=3  Side=Right
  - in : PMIOPort  Port=4  Side=Right
  wires:
  Voltage Measurement/1 -> Scope2/1
  Voltage Measurement3/1 -> Scope1/1
  Constant/1 -> PWM Generator (DC-DC)/1
  PWM Generator (DC-DC)/1 -> Mosfet/1
  connections:
  Voltage Measurement/LConn1 -- + out/RConn1 -- Series RLC Branch1/LConn1 -- Diode/RConn1
  Voltage Measurement3/LConn1 -- + in/RConn1 -- Series RLC Branch/LConn1
  Voltage Measurement/LConn2 -- - out/RConn1 -- Series RLC Branch1/RConn1 -- Voltage Measurement3/LConn2 -- - in/RConn1 -- Mosfet/RConn1
  Series RLC Branch/RConn1 -- Diode/LConn1 -- Mosfet/LConn1
